simulink library "amg_sense_light_lib"  (R2015b)
settings: Solver=ode45  StartTime=0.0  StopTime=10.0  RelTol=1e-3
libraries: simulink x37, stm32f4_i2c_lib x3, waijung_soft_i2c_lib x3, waijung_customcode x1
(part 2 of 2)

== system amg_sense_light_lib/APDS 9301/SCALE/Subsystem1/Subsystem ==
  In1 : Inport
  Enable : EnablePort  PropagateVarSize=During execution
  Bitwise Operator : simulink/Logic and Bit Operations/Bitwise Operator  logicop=AND  UseBitMask=on  BitMask=3  BitMaskRealWorld=Stored Integer
  Constant1 : Constant
  Constant2 : Constant  Value=0.034
  Constant3 : Constant  Value=0.252
  Multiport Switch : MultiPortSwitch  DataPortOrder=Zero-based contiguous  Inputs=4  zeroidx=on
  Out1 : Outport
  wires:
  Bitwise Operator/1 -> Multiport Switch/1
  In1/1 -> Bitwise Operator/1
  Constant2/1 -> Multiport Switch/2
  Constant3/1 -> Multiport Switch/3
  Constant1/1 -> Multiport Switch/4, Multiport Switch/5
  Multiport Switch/1 -> Out1/1
